simulink model "State_space_model_integrator_method"  (R2024a)
settings: Solver=VariableStepAuto  StartTime=0.0  StopTime=10.0  RelTol=1e-3
values from neighbouring files (symbols this model uses):
  b = 1    [State_space_parameters.mat]
  k = 5    [State_space_parameters.mat]
  m = 10    [State_space_parameters.mat]
settings Model: Creator=nassa  LastModifiedBy=nassa

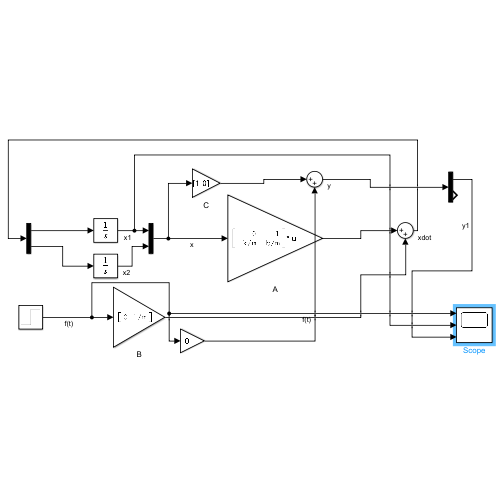
[thumbnail: Simulink's stored preview of the top-level diagram]
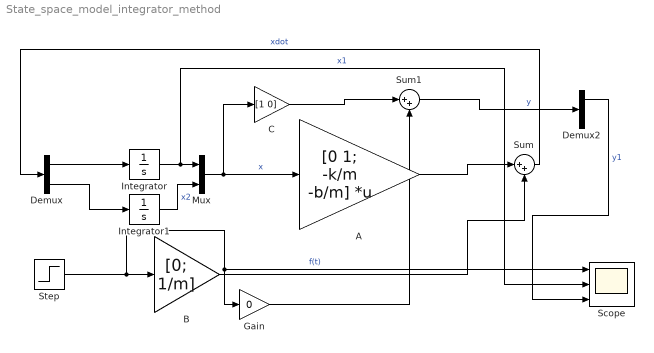
== system State_space_model_integrator_method ==
  A : Gain  Gain=[0 1; -k/m -b/m]  Multiplication=Matrix(K*u)
  B : Gain  Gain=[0; 1/m]
  C : Gain  Gain=[1 0]
  Demux : Demux  Outputs=2
  Demux2 : Demux  Outputs=2
  Gain : Gain  Gain=0
  Integrator : Integrator
  Integrator1 : Integrator
  Mux : Mux  Inputs=2
  Scope : Scope  NumInputPorts=3
  Step : Step  SampleTime=0
  Sum : Sum  Inputs=|++
  Sum1 : Sum  Inputs=|++
  wires:
  Step/1 -> Scope/1, Gain/1, B/1  "f(t)"
  A/1 -> Sum/1
  Demux/1 -> Integrator/1
  Demux/2 -> Integrator1/1
  Integrator1/1 -> Mux/2  "x2"
  Integrator/1 -> Scope/2, Mux/1  "x1"
  Mux/1 -> C/1, A/1  "x"
  Sum/1 -> Demux/1  "xdot"
  B/1 -> Sum/2
  C/1 -> Sum1/1
  Gain/1 -> Sum1/2
  Sum1/1 -> Demux2/1  "y"
  Demux2/1 -> Scope/3  "y1"
